simulink library "HANcoder_STM32_Target"  (R2018a)
settings: Solver=ode45  StartTime=0.0  StopTime=10.0  RelTol=1e-3  EnableMultiTasking=on
libraries: simulink x3
(part 1 of 7)
settings Model: Creator=HANcoder  LastModifiedBy=tatzs
settings Model: ModifiedHistory=|
  | la_obwlf -- Thu Sep 01 12:12:55 2016 -- Version 0.33
  | 
  | 
  | 
  | 
  | 
  | 
  | la_obwlf -- Thu Sep 01 09:23:34 2016 -- Version 0.33
  | changed the version in the Base Sample Time block
  | 
  | 
  | 
  | la_obwlf -- Tue Aug 30 15:48:17 2016 -- Version 0.33
settings DataIOCC: LimitDataPoints=on  SaveFormat=Array  SignalLoggingSaveFormat=ModelDataLogs
settings OptimizationCC: ExpressionDepthLimit=2147483647  LifeSpan=inf
settings DebuggingCC: UnderspecifiedInitializationDetection=Classic  MergeDetectMultiDrivingBlocksExec=none  SolverPrmCheckMsg=warning  FcnCallInpInsideContextMsg=warning  StateNameClashWarn=warning  SFUnexpectedBacktrackingDiag=warning  SFNoUnconditionalDefaultTransitionDiag=warning  SFExecutionAtInitializationDiag=none
settings HardwareCC: ProdBitPerPointer=32  ProdBitPerSizeT=32  ProdBitPerPtrDiffT=32  ProdLargestAtomicFloat=None  ProdIntDivRoundTo=Undefined  ProdEndianess=Unspecified  ProdWordSize=32  ProdHWDeviceType=32-bit Generic
settings ModelReferenceCC: PropagateSignalLabelsOutOfModel=off
settings CodeAppCC: StateflowObjectComments=on
settings GRTTargetCC: TargetLangStandard=C89/C90 (ANSI)  GeneratePreprocessorConditionals=Disable all  CombineOutputUpdateFcns=off  GRTInterface=on
settings ConfigComp: CovMetricSettings=dw  CovHtmlReporting=on  CovSaveCumulativeToWorkspaceVar=on  CovSaveSingleToWorkspaceVar=on  CovExternalEMLEnable=off

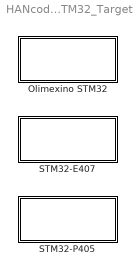
== system HANcoder_STM32_Target ==
  Olimexino STM32 : Subsystem
      settings: MoveFcn=drawLogos
      mask Display:
      | disp('Olimexino STM32')
      | patch([80 86 86],[8 14 2],[1 0 0]);patch([88 88 94],[14 2 8],[0 0 0.35]);
  STM32-E407 : Subsystem
      settings: MoveFcn=drawLogos
      mask Display:
      | disp('STM32-E407')
      | patch([80 86 86],[8 14 2],[1 0 0]);patch([88 88 94],[14 2 8],[0 0 0.35]);
  STM32-P405 : Subsystem
      settings: MoveFcn=drawLogos
      mask Display:
      | disp('STM32-P405')
      | patch([80 86 86],[8 14 2],[1 0 0]);patch([88 88 94],[14 2 8],[0 0 0.35]);

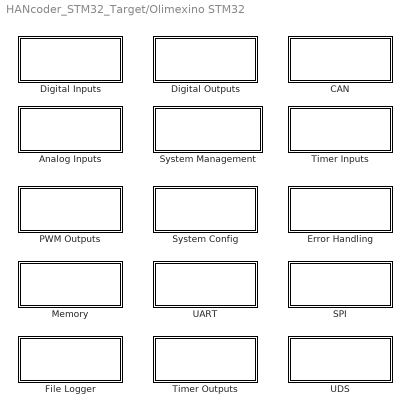
== system HANcoder_STM32_Target/Olimexino STM32 ==
  Analog Inputs : Subsystem
      settings: MoveFcn=drawLogos
      mask Display: fprintf('Analog Inputs');patch([85 91 91],[8 14 2],[1 0 0]);patch([93 93 99],[14 2 8],[0 0 0.35]);
  CAN : Subsystem
      settings: MoveFcn=drawLogos
      mask Display: fprintf('CAN');patch([85 91 91],[8 14 2],[1 0 0]);patch([93 93 99],[14 2 8],[0 0 0.35]);
  Digital Inputs : Subsystem
      settings: MoveFcn=drawLogos
      mask Display: fprintf('Digital Inputs');patch([85 91 91],[8 14 2],[1 0 0]);patch([93 93 99],[14 2 8],[0 0 0.35]);
  Digital Outputs : Subsystem
      settings: MoveFcn=drawLogos
      mask Display: fprintf('Digital Outputs');patch([85 91 91],[8 14 2],[1 0 0]);patch([93 93 99],[14 2 8],[0 0 0.35]);
  Error Handling : Subsystem
      settings: MoveFcn=drawLogos
      mask Display: fprintf('Error Handling');patch([85 91 91],[8 14 2],[1 0 0]);patch([93 93 99],[14 2 8],[0 0 0.35]);
  File Logger : Subsystem
      settings: MoveFcn=drawLogos
      mask Display: fprintf('File Logger');patch([85 91 91],[8 14 2],[1 0 0]);patch([93 93 99],[14 2 8],[0 0 0.35]);
  Memory : Subsystem
      settings: MoveFcn=drawLogos
      mask Display: fprintf('Memory');patch([85 91 91],[8 14 2],[1 0 0]);patch([93 93 99],[14 2 8],[0 0 0.35]);
  PWM Outputs : Subsystem
      settings: MoveFcn=drawLogos
      mask Display: fprintf('PWM Outputs');patch([85 91 91],[8 14 2],[1 0 0]);patch([93 93 99],[14 2 8],[0 0 0.35]);
  SPI : Subsystem
      settings: MoveFcn=drawLogos
      mask Display: fprintf('SPI');patch([85 91 91],[8 14 2],[1 0 0]);patch([93 93 99],[14 2 8],[0 0 0.35]);
  System Config : Subsystem  RequirementInfo={} %GIDa_b102142c_ec72_4a3a_aedf_acb717d0b820
      settings: MoveFcn=drawLogos
      mask Display: fprintf('System Config');patch([85 91 91],[8 14 2],[1 0 0]);patch([93 93 99],[14 2 8],[0 0 0.35]);
  System Management : Subsystem
      settings: MoveFcn=drawLogos
      mask Display: fprintf('System Management');patch([90 96 96],[8 14 2],[1 0 0]);patch([98 98 104],[14 2 8],[0 0 0.35]);
  Timer Inputs : Subsystem
      settings: MoveFcn=drawLogos
      mask Display: fprintf('Timer Inputs');patch([85 91 91],[8 14 2],[1 0 0]);patch([93 93 99],[14 2 8],[0 0 0.35]);
  Timer Outputs : Subsystem
      settings: MoveFcn=drawLogos
      mask Display: fprintf('Timer Outputs');patch([85 91 91],[8 14 2],[1 0 0]);patch([93 93 99],[14 2 8],[0 0 0.35]);
  UART : Subsystem
      settings: MoveFcn=drawLogos
      mask Display: fprintf('UART');patch([85 91 91],[8 14 2],[1 0 0]);patch([93 93 99],[14 2 8],[0 0 0.35]);
  UDS : Subsystem
      settings: MoveFcn=drawLogos
      mask Display: fprintf('UDS');patch([85 91 91],[8 14 2],[1 0 0]);patch([93 93 99],[14 2 8],[0 0 0.35]);

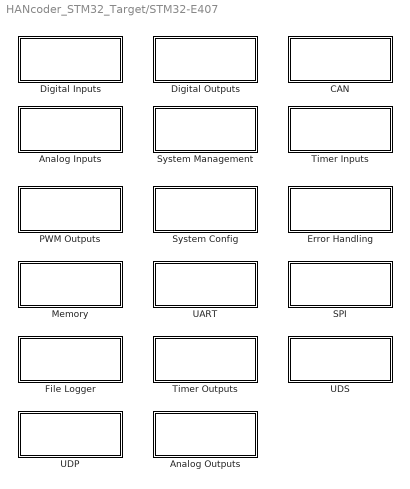
== system HANcoder_STM32_Target/STM32-E407 ==
  Analog Inputs : Subsystem
      settings: MoveFcn=drawLogos
      mask Display: fprintf('Analog Inputs');patch([85 91 91],[8 14 2],[1 0 0]);patch([93 93 99],[14 2 8],[0 0 0.35]);
  Analog Outputs : Subsystem
      settings: MoveFcn=drawLogos
      mask Display: fprintf('Analog Outputs');patch([85 91 91],[8 14 2],[1 0 0]);patch([93 93 99],[14 2 8],[0 0 0.35]);
  CAN : Subsystem
      settings: MoveFcn=drawLogos
      mask Display: fprintf('CAN');patch([85 91 91],[8 14 2],[1 0 0]);patch([93 93 99],[14 2 8],[0 0 0.35]);
  Digital Inputs : Subsystem
      settings: MoveFcn=drawLogos
      mask Display: fprintf('Digital Inputs');patch([85 91 91],[8 14 2],[1 0 0]);patch([93 93 99],[14 2 8],[0 0 0.35]);
  Digital Outputs : Subsystem
      settings: MoveFcn=drawLogos
      mask Display: fprintf('Digital Outputs');patch([85 91 91],[8 14 2],[1 0 0]);patch([93 93 99],[14 2 8],[0 0 0.35]);
  Error Handling : Subsystem
      settings: MoveFcn=drawLogos
      mask Display: fprintf('Error Handling');patch([85 91 91],[8 14 2],[1 0 0]);patch([93 93 99],[14 2 8],[0 0 0.35]);
  File Logger : Subsystem
      settings: MoveFcn=drawLogos
      mask Display: fprintf('File Logger');patch([85 91 91],[8 14 2],[1 0 0]);patch([93 93 99],[14 2 8],[0 0 0.35]);
  Memory : Subsystem
      settings: MoveFcn=drawLogos
      mask Display: fprintf('Memory');patch([85 91 91],[8 14 2],[1 0 0]);patch([93 93 99],[14 2 8],[0 0 0.35]);
  PWM Outputs : Subsystem
      settings: MoveFcn=drawLogos
      mask Display: fprintf('PWM Outputs');patch([85 91 91],[8 14 2],[1 0 0]);patch([93 93 99],[14 2 8],[0 0 0.35]);
  SPI : Subsystem
      settings: MoveFcn=drawLogos
      mask Display: fprintf('SPI');patch([85 91 91],[8 14 2],[1 0 0]);patch([93 93 99],[14 2 8],[0 0 0.35]);
  System Config : Subsystem  RequirementInfo={} %GIDa_b102142c_ec72_4a3a_aedf_acb717d0b820
      settings: MoveFcn=drawLogos
      mask Display: fprintf('System Config');patch([85 91 91],[8 14 2],[1 0 0]);patch([93 93 99],[14 2 8],[0 0 0.35]);
  System Management : Subsystem
      settings: MoveFcn=drawLogos
      mask Display: fprintf('System Management');patch([85 91 91],[8 14 2],[1 0 0]);patch([93 93 99],[14 2 8],[0 0 0.35]);
  Timer Inputs : Subsystem
      settings: MoveFcn=drawLogos
      mask Display: fprintf('Timer Inputs');patch([85 91 91],[8 14 2],[1 0 0]);patch([93 93 99],[14 2 8],[0 0 0.35]);
  Timer Outputs : Subsystem
      settings: MoveFcn=drawLogos
      mask Display: fprintf('Timer Outputs');patch([85 91 91],[8 14 2],[1 0 0]);patch([93 93 99],[14 2 8],[0 0 0.35]);
  UART : Subsystem
      settings: MoveFcn=drawLogos
      mask Display: fprintf('UART');patch([85 91 91],[8 14 2],[1 0 0]);patch([93 93 99],[14 2 8],[0 0 0.35]);
  UDP : Subsystem
      settings: MoveFcn=drawLogos
      mask Display: fprintf('UDP');patch([85 91 91],[8 14 2],[1 0 0]);patch([93 93 99],[14 2 8],[0 0 0.35]);
  UDS : Subsystem
      settings: MoveFcn=drawLogos
      mask Display: fprintf('UDS');patch([85 91 91],[8 14 2],[1 0 0]);patch([93 93 99],[14 2 8],[0 0 0.35]);

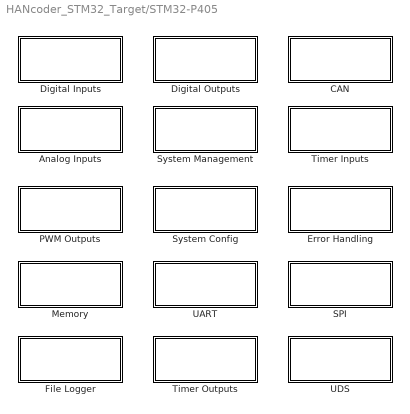
== system HANcoder_STM32_Target/STM32-P405 ==
  Analog Inputs : Subsystem
      settings: MoveFcn=drawLogos
      mask Display: fprintf('Analog Inputs');patch([85 91 91],[8 14 2],[1 0 0]);patch([93 93 99],[14 2 8],[0 0 0.35]);
  CAN : Subsystem
      settings: MoveFcn=drawLogos
      mask Display: fprintf('CAN');patch([85 91 91],[8 14 2],[1 0 0]);patch([93 93 99],[14 2 8],[0 0 0.35]);
  Digital Inputs : Subsystem
      settings: MoveFcn=drawLogos
      mask Display: fprintf('Digital Inputs');patch([85 91 91],[8 14 2],[1 0 0]);patch([93 93 99],[14 2 8],[0 0 0.35]);
  Digital Outputs : Subsystem
      settings: MoveFcn=drawLogos
      mask Display: fprintf('Digital Outputs');patch([85 91 91],[8 14 2],[1 0 0]);patch([93 93 99],[14 2 8],[0 0 0.35]);
  Error Handling : Subsystem
      settings: MoveFcn=drawLogos
      mask Display: fprintf('Error Handling');patch([85 91 91],[8 14 2],[1 0 0]);patch([93 93 99],[14 2 8],[0 0 0.35]);
  File Logger : Subsystem
      settings: MoveFcn=drawLogos
      mask Display: fprintf('File Logger');patch([85 91 91],[8 14 2],[1 0 0]);patch([93 93 99],[14 2 8],[0 0 0.35]);
  Memory : Subsystem
      settings: MoveFcn=drawLogos
      mask Display: fprintf('Memory');patch([85 91 91],[8 14 2],[1 0 0]);patch([93 93 99],[14 2 8],[0 0 0.35]);
  PWM Outputs : Subsystem
      settings: MoveFcn=drawLogos
      mask Display: fprintf('PWM Outputs');patch([85 91 91],[8 14 2],[1 0 0]);patch([93 93 99],[14 2 8],[0 0 0.35]);
  SPI : Subsystem
      settings: MoveFcn=drawLogos
      mask Display: fprintf('SPI');patch([85 91 91],[8 14 2],[1 0 0]);patch([93 93 99],[14 2 8],[0 0 0.35]);
  System Config : Subsystem  RequirementInfo={} %GIDa_b102142c_ec72_4a3a_aedf_acb717d0b820
      settings: MoveFcn=drawLogos
      mask Display: fprintf('System Config');patch([85 91 91],[8 14 2],[1 0 0]);patch([93 93 99],[14 2 8],[0 0 0.35]);
  System Management : Subsystem
      settings: MoveFcn=drawLogos
      mask Display: fprintf('System Management');patch([85 91 91],[8 14 2],[1 0 0]);patch([93 93 99],[14 2 8],[0 0 0.35]);
  Timer Inputs : Subsystem
      settings: MoveFcn=drawLogos
      mask Display: fprintf('Timer Inputs');patch([85 91 91],[8 14 2],[1 0 0]);patch([93 93 99],[14 2 8],[0 0 0.35]);
  Timer Outputs : Subsystem
      settings: MoveFcn=drawLogos
      mask Display: fprintf('Timer Outputs');patch([85 91 91],[8 14 2],[1 0 0]);patch([93 93 99],[14 2 8],[0 0 0.35]);
  UART : Subsystem
      settings: MoveFcn=drawLogos
      mask Display: fprintf('UART');patch([85 91 91],[8 14 2],[1 0 0]);patch([93 93 99],[14 2 8],[0 0 0.35]);
  UDS : Subsystem
      settings: MoveFcn=drawLogos
      mask Display: fprintf('UDS');patch([85 91 91],[8 14 2],[1 0 0]);patch([93 93 99],[14 2 8],[0 0 0.35]);

== system HANcoder_STM32_Target/Olimexino STM32/Analog Inputs ==
  Analog Input : Subsystem  Tag=HANcoder_TARGET_STM32_Olimexino  mask(Analog Input){pinID=CON2 - A0, tsamp=-1, filtered=off}
      mask prompts: pinID "Input pin"; tsamp "Sample time"; filtered "Use oversampling and filtering (causes high CPU load)"
      mask help:
      | Function
      | ========
      | Reads the analog/digital conversion results of an analog input pin.
      |
      | Parameters
      | ==========
      | Input pin:
      |   Selects the analog input to read
      |
      | Outport
      | ==========
      | uint16 12-bit conversion results (0-4095).
      mask init:
      | pinIDInfoStr = sfcn_analog_in_mcb(1, pinID, 0);
      settings: MoveFcn=drawLogos
      mask Help: web('sfcn_analog_in.html');
      mask TypeOptions pinID: CON2 - A0 | CON2 - A1 | CON2 - A2 | CON2 - A3 | CON2 - A4 | CON2 - A5 | CON3 - D0 | CON3 - D1 | CON3 - D2 | CON3 - D3/LED2 | CON4 - D10 | CON4 - D11 | CON4 - D12 | CON4 - D13/LED1 | EXT - D27 | EXT - D28
      mask Display: fprintf('Analog Input\n%s', pinIDInfoStr);patch([135 141 141],[8 14 2],[1 0 0]);patch([143 143 149],[14 2 8],[0 0 0.35]);

== system HANcoder_STM32_Target/Olimexino STM32/CAN ==
  CAN : Subsystem
      settings: MoveFcn=drawLogos
      mask Display: fprintf('CAN');patch([85 91 91],[8 14 2],[1 0 0]);patch([93 93 99],[14 2 8],[0 0 0.35]);
  CANopenClient : Subsystem
      settings: MoveFcn=drawLogos
      mask Display: fprintf('CANopenClient');patch([85 91 91],[8 14 2],[1 0 0]);patch([93 93 99],[14 2 8],[0 0 0.35]);
  CANopenNode : Subsystem
      settings: MoveFcn=drawLogos
      mask Display: fprintf('CANopenNode');patch([85 91 91],[8 14 2],[1 0 0]);patch([93 93 99],[14 2 8],[0 0 0.35]);

== system HANcoder_STM32_Target/Olimexino STM32/Digital Inputs ==
  Digital Input : Subsystem  Tag=HANcoder_TARGET_STM32_Olimexino  mask(Digital Input){pinID=CON2 - A0, config=Pulldown, tsamp=-1}
      mask prompts: pinID "Input pin"; config "Configuration"; tsamp "Sample time"
      mask help:
      | Function
      | ========
      | Reads the state of a digital input pin.
      |
      | Parameters
      | ==========
      | Input pin:
      |   Selects the digital input to read
      | Configuration:
      |   Determines if the input is floating or is connected to an internal
      |   pull-up or pull-down resistor.
      |
      | Outport
      | ==========
      | State of the pin. 0 means logical low and 1 logical high
      mask init:
      | pinIDInfoStr = sfcn_digital_in_mcb(1, pinID, config);
      settings: MoveFcn=drawLogos
      mask Help: web('sfcn_digital_in.html');
      mask TypeOptions pinID: CON2 - A0 | CON2 - A1 | CON2 - A2 | CON2 - A3 | CON2 - A4 | CON2 - A5 | CON3 - D0 | CON3 - D1 | CON3 - D2 | CON3 - D3/LED2 | CON3 - D4 | CON3 - D5 - 5V Tolerant | CON3 - D6 - 5V Tolerant | CON3 - D7 - 5V Tolerant | CON4 - D8 - 5V Tolerant | CON4 - D9 - 5V Tolerant | CON4 - D10 | CON4 - D11 | CON4 - D12 | CON4 - D13/LED1 | EXT - D25 - 5V Tolerant | EXT - D26 - 5V Tolerant | EXT - D29 - 5V Tolerant | EXT - D30 - 5V Tolerant | EXT - D31 - 5V Tolerant | EXT - D32 - 5V Tolerant | EXT - D33 - 5V Tolerant | EXT - D34 - 5V Tolerant | EXT - D35 - 5V Tolerant | EXT - D36 - 5V Tolerant | EXT - D37 - 5V Tolerant | Pushbutton - BUT/BOOT0 - 5V Tolerant
      mask TypeOptions config: Floating | Pullup | Pulldown
      mask Display: fprintf('Digital Input\n%s', pinIDInfoStr);patch([135 141 141],[8 14 2],[1 0 0]);patch([143 143 149],[14 2 8],[0 0 0.35]);

== system HANcoder_STM32_Target/Olimexino STM32/Digital Outputs ==
  Digital Output : Subsystem  Tag=HANcoder_TARGET_STM32_Olimexino  mask(Digital Output){pinID=CON2 - A0, config=Push pull, tsamp=-1}
      mask prompts: pinID "Output pin"; config "Configuration"; tsamp "Sample time"
      mask help:
      | Function
      | ========
      | Controls the state of a digital output pin.
      |
      | Parameters
      | ==========
      | Output pin:
      |   Selects the digital output to control
      | Configuration:
      |   Open drain (output float when digital high) or push-pull (output connected
      |   to Vcc when digital high).
      |
      | Inport
      | ==========
      | State of the pin. 0 means logical low and 1 logical high
      mask init:
      | pinIDInfoStr = sfcn_digital_out_mcb(1, pinID, config);
      settings: CopyFcn=sfcn_digital_out_chk();  MoveFcn=drawLogos
      mask Help: web('sfcn_digital_out.html');
      mask TypeOptions pinID: CON2 - A0 | CON2 - A1 | CON2 - A2 | CON2 - A3 | CON2 - A4 | CON2 - A5 | CON3 - D0 | CON3 - D1 | CON3 - D2 | CON3 - D3/LED2 | CON3 - D4 | CON3 - D5 | CON3 - D6 | CON3 - D7 | CON4 - D8 | CON4 - D9 | CON4 - D10 | CON4 - D11 | CON4 - D12 | CON4 - D13/LED1 | EXT - D25 | EXT - D26 | EXT - D31 | EXT - D32 | EXT - D35 | EXT - D36 | EXT - D37
      mask Callback pinID: sfcn_digital_out_chk();
      mask TypeOptions config: Open drain | Push pull
      mask Display: fprintf('Digital Output\n%s', pinIDInfoStr);patch([135 141 141],[8 14 2],[1 0 0]);patch([143 143 149],[14 2 8],[0 0 0.35]);

== system HANcoder_STM32_Target/Olimexino STM32/Error Handling ==
  Clear errors : Subsystem  Tag=HANcoder_TARGET_STM32_Olimexino  mask(Clear errors){eepromString=Active}
      mask prompts: eepromString "Active or Stored error"
      mask help:
      | [Function]
      | Clears the active(RAM) or stored(EEPROM) errors.
      |
      | [Triggerport]
      | Connect the port to a trigger source to execute the block only when necessary.
      mask init:
      | sfcn_controller_error_clearerrors_mcb(eepromString)
      settings: MoveFcn=drawLogos
      mask Help: web('sfcn_controller_error_clearerrors.html');
      mask TypeOptions eepromString: Active | Stored
      mask Display: fprintf('Clear %s Errors', eepromString);patch([80 86 86],[8 14 2],[1 0 0]);patch([88 88 94],[14 2 8],[0 0 0.35]);
  Delete error : Subsystem  Tag=HANcoder_TARGET_STM32_Olimexino  mask(Delete error){useInPorts=off, errorID=hex2dec('8000'), para=10}
      mask prompts: useInPorts "Use inports"; errorID "Error code"; para "Error parameter"
      mask help:
      | [Function]
      | Delete an error defined by error code and parameter
      | from RAM.
      | Error ID and parameter can be specified in the mask or with inports.
      |
      | [Parameters]
      | Error code
      | Error parameter
      |
      | [Inputs]
      | 1 - Error code [uint16]
      | 2 - Error parameter [uint8]
      |
      | [Triggerport]
      | Connect the port to a trigger source to execute the block only when necessary.
      mask init:
      | sfcn_controller_error_deleteerror_mcb(useInPorts, errorID, para)
      settings: MoveFcn=drawLogos
      mask Help: web('sfcn_controller_error_deleteerror.html');
      mask Display: fprintf('Delete error');patch([80 86 86],[8 14 2],[1 0 0]);patch([88 88 94],[14 2 8],[0 0 0.35]);
  Read active error : Subsystem  Tag=HANcoder_TARGET_STM32_Olimexino  mask(Read active error){tsamp=-1}
      mask prompts: tsamp "Sample time"
      mask help:
      | Function
      | ==========
      | Read an active error from RAM.
      |
      | Inport
      | ==========
      | Input is the number of the error in the error list, which can be 1..64. UINT8
      |
      | Outports
      | ==========
      | 1: UINT8 - total amount of errors.
      | 2: UINT16 - error code.
      | 3: UINT8  - error parameter.
      | 4: UINT8  - occurrence count.
      | 5: UINT32 - last occurrence time since startup [milliseconds].
      |
      | Note that the requested error was set and read only if occurrence count > 0.
      mask init:
      | sfcn_controller_error_readerror_mcb(0)
      settings: MoveFcn=drawLogos
      mask Help: web('sfcn_controller_error_readerror.html');
      mask Display: fprintf('Read active error');patch([80 86 86],[8 14 2],[1 0 0]);patch([88 88 94],[14 2 8],[0 0 0.35]);
  Read stored error : Subsystem  Tag=HANcoder_TARGET_STM32_Olimexino  mask(Read stored error){tsamp=-1}
      mask prompts: tsamp "Sample time"
      mask help:
      | Function
      | ==========
      | Read a stored error from EEPROM.
      |
      | Inport
      | ==========
      | Input is the number of the error in the error list, which can be 1..64. UINT8
      |
      | Outports
      | ==========
      | 1: UINT8 - total amount of errors.
      | 2: UINT16 - error code.
      | 3: UINT8  - error parameter.
      | 4: UINT8  - occurrence count.
      | 5: UINT32 - last occurrence time since startup [milliseconds].
      |
      | Note that the requested error was set and read only if occurrence count > 0.
      mask init:
      | sfcn_controller_error_readerror_mcb(1)
      settings: MoveFcn=drawLogos
      mask Help: web('sfcn_controller_error_readerror.html');
      mask Display: fprintf('Read stored error');patch([80 86 86],[8 14 2],[1 0 0]);patch([88 88 94],[14 2 8],[0 0 0.35]);
  Search active error : Subsystem  Tag=HANcoder_TARGET_STM32_Olimexino  mask(Search active error){tsamp=-1}
      mask prompts: tsamp "Sample time"
      mask help:
      | Function
      | ==========
      | Searches for the erorr with the specified error Code and Param in RAM.
      |
      | Inport
      | ==========
      | 1: UINT16 - Error Code
      | 2: UINT8   - Error Parameter
      |
      | Outports
      | ==========
      | 1: UINT8   - occurrence count.
      | 2: UINT32 - last occurrence time since startup [milliseconds]
      |
      | Note that when occurrence count equals zero, the error is not found.
      mask init:
      | sfcn_controller_error_searcherror_mcb(0)
      settings: MoveFcn=drawLogos
      mask Help: web('sfcn_controller_error_searcherror.html');
      mask Display: fprintf('Search active error');patch([80 86 86],[8 14 2],[1 0 0]);patch([88 88 94],[14 2 8],[0 0 0.35]);
  Search stored error : Subsystem  Tag=HANcoder_TARGET_STM32_Olimexino  mask(Search stored error){tsamp=-1}
      mask prompts: tsamp "Sample time"
      mask help:
      | Function
      | ==========
      | Searches for the erorr with the specified error Code and Param in EEPROM.
      |
      | Inport
      | ==========
      | 1: UINT16 - Error Code
      | 2: UINT8   - Error Parameter
      |
      | Outports
      | ==========
      | 1: UINT8   - occurrence count.
      | 2: UINT32 - last occurrence time since startup [milliseconds]
      |
      | Note that when occurrence count equals zero, the error is not found.
      mask init:
      | sfcn_controller_error_searcherror_mcb(1)
      settings: MoveFcn=drawLogos
      mask Help: web('sfcn_controller_error_searcherror.html');
      mask Display: fprintf('Search stored error');patch([80 86 86],[8 14 2],[1 0 0]);patch([88 88 94],[14 2 8],[0 0 0.35]);
  "Store error " : Subsystem  Tag=HANcoder_TARGET_STM32_Olimexino  mask(Store error){useInPorts=off, errorCode=hex2dec('8000'), parameter=10}
      mask prompts: useInPorts "Use inports"; errorCode "Error code"
      mask help:
      | [Function]
      | Store an error to RAM (and EEPROM if new) of the controller.
      | Error ID and parameter can be specified in the mask or with inports.
      |
      | [Parameters]
      | Error code
      | Error parameter
      |
      | [Inputs]
      | 1 - Error code [uint16]
      | 2 - Error parameter [uint8]
      |
      | [Triggerport]
      | Connect the port to a trigger source to execute the block only when necessary.
      mask init:
      | sfcn_controller_error_storeerror_in_mcb(useInPorts, errorCode, parameter, 1)
      settings: MoveFcn=drawLogos
      mask Help: web('sfcn_controller_error_storeerror.html');
      mask Display: fprintf('Store error');patch([80 86 86],[8 14 2],[1 0 0]);patch([88 88 94],[14 2 8],[0 0 0.35]);
  Total Errors : Subsystem  Tag=HANcoder_TARGET_STM32_Olimexino  mask(Total active or stored errors){eepromString=Active, tsamp=-1}
      mask prompts: eepromString "Active or Stored error"; tsamp "Sample time"
      mask help:
      | [Function]
      | Returns the total amount of active or stored errors
      |
      | [Parameters]
      | Active or Stored error [-]
      | sampleTime: [s]
      |
      | [Outputs]
      | Port 1 :Total number of errors [uint8]
      | Port 2 :Highest occuring severity [uint8]
      mask init:
      | sfcn_controller_error_totalerrors_mcb(eepromString, tsamp);
      settings: MoveFcn=drawLogos
      mask Help: web('sfcn_controller_error_totalerrors.html');
      mask TypeOptions eepromString: Active | Stored
      mask Display: fprintf('Total %s Errors', eepromString);patch([80 86 86],[8 14 2],[1 0 0]);patch([88 88 94],[14 2 8],[0 0 0.35]);

== system HANcoder_STM32_Target/Olimexino STM32/File Logger ==
  File Logger Close : Subsystem  Tag=HANcoder_TARGET_STM32_Olimexino  mask(File Logger Close){}
      mask help:
      | Function
      | ========
      | With the File Logger module active, the data values of the configured signals
      | are sampled at a fixed time interval and written to the log-file on the SD-card.
      |
      | The log-file needs to be explicitly closed at the end of a logging session for the
      | log-file to actually appear on the SD-card.
      |
      | Ideally, this block is called during software shutdown for example when the ignition
      | signal goes low in automotive applications. An external trigger can also be used such
      | as a button press event or CAN message reception.
      |
      | Triggerport
      | ===========
      | Connect the port to a trigger source to execute the block only when necessary.
      mask init:
      | sfcn_filelogger_close_mcb();
      settings: MoveFcn=drawLogos
      mask Help: web('sfcn_filelogger_close.html')
      mask Display: fprintf('File Logger Close');patch([80 86 86],[8 14 2],[1 0 0]);patch([88 88 94],[14 2 8],[0 0 0.35]);
  File Logger Init : Subsystem  Tag=HANcoder_TARGET_STM32_Olimexino  mask(File Logger Init){filename='mylog.txt', autoincrement=on, firstline='time;signal1;signal2;signal3', interval=100, maxsignals=3, dotseparator=off, autostart=on}
      mask prompts: autoincrement "Add auto-incrementing number to filename"; firstline "First line in log-file"; interval "Logging interval (ms)"; maxsignals "Maximum signals to log"; dotseparator "Use dot-character as decimal separator (comma otherwise)"; autostart "Automatically start logging"
      mask help:
      | Function
      | ==========
      | Initializes the File Logger module.
      |
      | Parameters per channel
      | ======================
      | - Specify filename for the log-file
      | - Select if a 3-digit auto-incrementing number should be added to the log-file
      | - Specify the first line in the log-file
      | - Specify the logging interval in milliseconds
      | - Specify the maximum number of signals to log
      | - Select if a comma or dot should be used a the decimal point in numbers
      | - Select if logging should automatically start after initialization. If not then
      |   a trigger input will appear that can be used to trigger the logging start.
      mask init:
      | sfcn_filelogger_init_mcb(filename, firstline, interval, maxsignals, dotseparator, autoincrement, autostart);
      settings: MoveFcn=drawLogos
      mask Help: web('sfcn_filelogger_init.html')
      mask Display: fprintf('File Logger Init');patch([95 101 101],[8 14 2],[1 0 0]);patch([103 103 109],[14 2 8],[0 0 0.35]);
  File Logger Signal : Subsystem  Tag=HANcoder_TARGET_STM32_Olimexino  mask(File Logger Signal){signalIdx=0, dataType=uint8}
      mask prompts: signalIdx "Signal Index"; dataType "Signal Data Type"
      mask help:
      | Function
      | ==========
      | Configures the signal to be logged by the File Logger module.
      |
      | Parameters per channel
      | ======================
      | - Specify the zero based index of the signal for the File Logger module. In the
      |   File Logger Init block the maximum number of signals was configured
      |   (max_signals). Valid values for this paramter are 0..(max_signals-1).
      | - Select the data type of the signal.
      mask init:
      | sfcn_filelogger_signal_mcb(signalIdx, dataType);
      settings: MoveFcn=drawLogos
      mask Help: web('sfcn_filelogger_signal.html')
      mask TypeOptions dataType: double | single | int8 | uint8 | int16 | uint16 | int32 | uint32
      mask Display: fprintf('File Logger Signal\n(Index %d)', signalIdx);patch([95 101 101],[8 14 2],[1 0 0]);patch([103 103 109],[14 2 8],[0 0 0.35]);

== system HANcoder_STM32_Target/Olimexino STM32/Memory ==
  EEPROM : Subsystem
      settings: MoveFcn=drawLogos
      mask Display: fprintf('EEPROM');patch([85 91 91],[8 14 2],[1 0 0]);patch([93 93 99],[14 2 8],[0 0 0.35]);

== system HANcoder_STM32_Target/Olimexino STM32/PWM Outputs ==
  PWM Duty Cycle : Subsystem  Tag=HANcoder_TARGET_STM32_Olimexino  mask(Pulse Width Modulation Set Duty Cycle){pinID=TIM1 - CON3 - D6, tsamp=-1}
      mask prompts: pinID "Output pin"; tsamp "Sample time"
      mask help:
      | Function
      | ========
      | A 'PWM Duty Cycle' block allows the duty cycle of the generated PWM signal to
      | changed.
      | Note that this only works properly if a 'PWM Init' block is also present
      | for initializing the related PWM module.
      |
      | Parameters
      | ==========
      | PWM pin:
      |   Selects the PWM pin for which the duty cycle should be updated.
      |
      | Inport
      | ==========
      | uint16 10-bit unsigned value (0..1023) to represent the duty cycle (0..100%) for
      | each enabled channel.
      mask init:
      | pinIDInfoStr = sfcn_pwmout_setduty_mcb(1, pinID);
      settings: MoveFcn=drawLogos
      mask Help: web('sfcn_pwmout_setduty.html');
      mask TypeOptions pinID: TIM1 - CON3 - D6 | TIM1 - CON3 - D7 | TIM1 - CON4 - D8 | TIM2 - CON3 - D2 | TIM2 - CON3 - D3 | TIM2 - CON3 - D0 | TIM3 - EXT - D35 | TIM3 - EXT - D36 | TIM3 - EXT - D37 | TIM4 - CON3 - D5 | TIM4 - CON4 - D9 | TIM4 - CON4 - D14 | TIM4 - EXT - D24
      mask Display: fprintf('PWM Set Duty Cycle\n%s', pinIDInfoStr);patch([135 141 141],[8 14 2],[1 0 0]);patch([143 143 149],[14 2 8],[0 0 0.35]);
  PWM Init : Subsystem  Tag=HANcoder_TARGET_STM32_Olimexino  mask(Pulse Width Modulation Initialization){moduleID=TIM1: D6 & D7 & D8 & n/a + N-channels D32 & D33 & D34, frequency=1004, alignment=Edge aligned, enableIRQoutput=off, ch1On=off, ch1Pol=Active high, ch1Inv=off, ch2On=off, ch2Pol=Active high, ch2Inv=off, ch3On=off, ch3Pol=Active high, ch3Inv=off, ch4On=off, ch4Pol=Active high, ch4Inv=off}
      mask prompts: moduleID "PWM module"; frequency "Signal frequency [Hz]"; alignment "Signal alignment"; enableIRQoutput "Enable IRQ output"; ch1On "Generate PWM signal on channel 1"; ch1Pol "Select signal polarity"; ch1Inv "Enable inverted signal on additional output pin"; ch2On "Generate PWM signal on channel 2"; ch2Pol "Select signal polarity"; ch2Inv "Enable inverted signal on additional output pin"; ch3On "Generate PWM signal on channel 3"; ch3Pol "Select signal polarity"; ch3Inv "Enable inverted signal on additional output pin"; ch4On "Generate PWM signal on channel 4"; ch4Pol "Select signal polarity"; ch4Inv "Enable inverted signal on additional output pin"
      mask help:
      | Function
      | ========
      | A 'PWM Init' block configures one of the STM32 timer modules for PWM
      | functionality, allowing a PWM signal to be generated on up to 4 timer
      | channels and their associated output pins.
      |
      | Parameters
      | ==========
      | General - PWM module:
      |   Select the PWM module to use. The name in the combo box contains
      |   information about which pins on the target belong to this timer module.
      |   Also the first pin corresponds with the first channel and so on:
      |   TIMx: Ch1 & Ch2 & Ch3...
      |
      | General - Signal frequency:
      |   Determines the signal frequency in Hz. If you click 'Apply' after entering
      |   the desired frequency it will automatically be adjusted to the closest
      |   supported value.
      |
      | General - Signal Aligment:
      |   Determines the aligment of the signal. It can either be edge aligned or
      |   center aligned.
      |
      | General - Enable IRQ output
      |   Controls whether or not the IRQ output is available.
      |
      | Channel x - Generate PWM signal on channel x:
      |   Enable to configure the channel for PWM functionality so that the PWM signal
      |   is outputted on the channel's associated microcontroller pin.
      |
      | Channel x - Signal polarity:
      |   Selects the polarity of the signal.
      |
      | Channel x - Enable inverted signal on additional output pin:
      |   When enabled, a second PWM signal will be generated on an additional
      |   microcontroller pin where the signal is an exact inversion of the first signal.
      mask init:
      | moduleIDInfoStr = sfcn_pwmout_init_mcb(1, moduleID, frequency, alignment, enableIRQoutput, ch1On, ch2On, ch3On, ch4On, ch1Pol, ch2Pol, ch3Pol, ch4Pol, ch1Inv, ch2Inv, ch3Inv, ch4Inv);
      settings: CopyFcn=sfcn_pwmout_init_chk();  MoveFcn=drawLogos
      mask Help: web('sfcn_pwmout_init.html');
      mask TypeOptions moduleID: TIM1: D6 & D7 & D8 & n/a + N-channels D32 & D33 & D34  | TIM2: D2 & D3 & n/a & D0 | TIM3: D35 & D36 & D37 & n/a | TIM4: D5 & D9 & D14 & D24
      mask Callback moduleID: sfcn_pwmout_init_chk();
      mask TypeOptions alignment: Edge aligned | Center aligned
      mask TypeOptions ch1Pol: Active high | Active low
      mask TypeOptions ch2Pol: Active high | Active low
      mask TypeOptions ch3Pol: Active high | Active low
      mask TypeOptions ch4Pol: Active high | Active low
      mask Display: fprintf('PWM Init\n%s', moduleIDInfoStr);patch([220 226 226],[8 14 2],[1 0 0]);patch([228 228 234],[14 2 8],[0 0 0.35]);

== system HANcoder_STM32_Target/Olimexino STM32/SPI ==
  SPI master init : Subsystem  Tag=HANcoder_TARGET_STM32_Olimexino  mask(SPI master init){channel=SPI1: D13 & D12 & D11, speed=9000 kHz, polarity=Idle low, phase=Sample bit on 1st clock edge}
      mask prompts: speed "Communication speed"
      mask help:
      | Function
      | ==========
      | Initialized a SPI master channel.
      |
      | Parameters per channel
      | ======================
      | - Select channel (SCK MISO MOSI)
      | - Select communication speed
      | - Select clock signal polarity
      | - Select clock phase to sample a bit
      mask init:
      | spiChannelInfoStr = sfcn_spi_master_init_mcb(1, channel, speed, polarity, phase);
      settings: CopyFcn=sfcn_spi_master_init_chk();  MoveFcn=drawLogos
      mask Help: web('sfcn_spi_master_init.html')
      mask TypeOptions channel: SPI1: D13 & D12 & D11 | SPI2: D32 & D33 & D34
      mask Callback channel: sfcn_spi_master_init_chk();
      mask TypeOptions speed: 36000 kHz | 18000 kHz | 9000 kHz | 4500 kHz | 2250 kHz | 1125 kHz | 562.5 kHz | 281.25 kHz
      mask TypeOptions polarity: Idle low | Idle high
      mask TypeOptions phase: Sample bit on 1st clock edge | Sample bit on 2nd clock edge
      mask Display: fprintf('SPI master init\n%s', spiChannelInfoStr);patch([211 217 217],[8 14 2],[1 0 0]);patch([219 219 225],[14 2 8],[0 0 0.35]);
  SPI master transfer : Subsystem  Tag=HANcoder_TARGET_STM32_Olimexino  mask(SPI master transfer){channel=SPI1: D13 & D12 & D11, useSS=off, SSpin=CON2 - A0, SSenable=on, SSdisable=on, delayCycles=0, tsamp=-1}
      mask prompts: useSS "Use slave select output"; SSpin "Slave select output pin"; SSenable "Enable slave select before transfer"; SSdisable "Disable slave select after transfer"; delayCycles "Delay cycles between slave select enable and transfer"; tsamp "Sample time"
      mask help:
      | Function
      | ==========
      | Performs a byte transfer via SPI.
      |
      | Parameters per channel
      | ======================
      | - Select channel
      | - Select if a Slave Select output should be controlled
      |   * Select the Slave Select digital output pin
      |   * Select if the Slave Select should be made logic low before the transfer
      |   * Select if the Slave Select should be made logic high after the transfer
      |   * Enter the number of CPU cycles to delay between Slave Select enable and the transfer
      |
      | Inputs
      | ======
      | The byte value to send to the slave.
      |
      | Outputs
      | =======
      | The byte value received from the slave.
      mask init:
      | spiChannelInfoStr = sfcn_spi_master_transfer_mcb(1, channel, useSS, SSpin, SSenable, SSdisable, delayCycles);
      settings: MoveFcn=drawLogos
      mask Help: web('sfcn_spi_master_transfer.html')
      mask TypeOptions channel: SPI1: D13 & D12 & D11 | SPI2: D32 & D33 & D34
      mask TypeOptions SSpin: CON2 - A0 | CON2 - A1 | CON2 - A2 | CON2 - A3 | CON2 - A4 | CON2 - A5 | CON3 - D0 | CON3 - D1 | CON3 - D2 | CON3 - D3/LED2 | CON3 - D4 | CON3 - D5 | CON3 - D6 | CON3 - D7 | CON4 - D8 | CON4 - D9 | CON4 - D10 | CON4 - D11 | CON4 - D12 | CON4 - D13/LED1 | EXT - D25 | EXT - D26 | EXT - D31 | EXT - D32 | EXT - D35 | EXT - D36 | EXT - D37
      mask Display: fprintf('SPI master transfer\n%s', spiChannelInfoStr);patch([210 216 216],[8 14 2],[1 0 0]);patch([218 218 224],[14 2 8],[0 0 0.35]);

== system HANcoder_STM32_Target/Olimexino STM32/System Config ==
  Base Sample Time config : Subsystem  Tag=HANcoder_TARGET_STM32_Olimexino  Description=HANcoder Target STM32-Olimexino blockset version 0.5  mask(Base Sample Time config){baseSampleTime=10, extraStack=25}
      mask prompts: baseSampleTime "Define the base sample time [ms]"; extraStack "Additional task stack (bytes):"
      mask help:
      | Function
      | ==========
      | Sets the Base Sample Time in the model, and automatically sets the sample
      | time in the solver step time menu when the model is simulated or build.
      |
      | Parameters
      | ==========
      | Base Sample Time [milliseconds]
      | Default:    10[ms]
      | Min:        0.1[ms]
      |
      | Note: This is the only block where sample time is set in miliseconds,
      | all other blocks work with sample time in seconds
      |
      | It is possible to reserve extra stack space for the OS task that executes
      | the model on the embedded target (AppCtrlTask).
      mask init:
      | sfcn_base_sample_time_mcb(baseSampleTime*1000, extraStack,1);
      | HANcoderStruct = get_param(gcb,'UserData');
      | BlocksetVersion = HANcoderStruct.BlocksetVersion;
      settings: MoveFcn=drawLogos
      mask Help: web('sfcn_base_sample_time.html')
      mask Display: fprintf('Blockset version %s\nBase Sample Time:\n %gms',BlocksetVersion,baseSampleTime);patch([91 97 97],[8 14 2],[1 0 0]);patch([99 99 105],[14 2 8],[0 0 0.35]);
  Build settings : Subsystem  Tag=HANcoder_TARGET_STM32_Olimexino  mask(Build Settings){AutoASAP2add=on, AutoFlash=USB}
      mask prompts: AutoASAP2add "Add signals and parameters automatically"; AutoFlash "Automatic flash after build"
      mask help:
      | Function
      | ==========
      | Auto Add:
      | Here you can turn the automatic adding of Signals and Parameters on or off. If the option is on all the parameters and signals which are not defined in the workspace will be added. You will be prompted for the value.
      |
      | Auto Flash:
      | This option will automatically start MicroBoot with the selected interface.
      settings: MoveFcn=drawLogos
      mask Help: web('build_settings.html')
      mask TypeOptions AutoASAP2add: on | off
      mask TypeOptions AutoFlash: off | USB | CAN
      mask DialogControl ParameterTabVar0 Prompt: Auto Add
      mask DialogControl Control3 Prompt: With this option the undefined parameters and signals will automatically be added to the workspace for use with HANtune. You will be prompted for the parameter values.
      mask DialogControl ParameterTabVar01 Prompt: Auto Flash
      mask DialogControl Control2 Prompt: With this option you can choose to automatically start MicroBoot after the build is complete. MicroBoot will start flashing using the selected interface.
      mask Display: fprintf('Build settings\nAuto Add: %s\nAuto Flash: %s',AutoASAP2add, AutoFlash);patch([114 120 120],[8 14 2],[1 0 0]);patch([122 122 128],[14 2 8],[0 0 0.35]);
  CAN config : Subsystem  Tag=HANcoder_TARGET_STM32_Olimexino  mask(CAN config){canBus1=on, baudRate1=500, rxMask1=hex2dec('00000000'), rxCode1=hex2dec('00000000'), rxMode1=Receive only 11-bit message identifiers, txBufSize1=32, evBufSize1=32}
      mask prompts: canBus1 "Use CAN bus"; baudRate1 "Baudrate CAN bus [kbit/s]"; rxMask1 "Reception filter Mask CAN bus"; rxCode1 "Reception filter Code CAN bus"; rxMode1 "Reception filter Mode CAN bus"; txBufSize1 "Transmit buffer size CAN bus (max 256)"; evBufSize1 "Event buffer size CAN bus"
      mask help:
      | Function
      | ==========
      | Configures the settings for the STM32's CAN busses.
      |
      | Parameters per channel
      | ======================
      | - Activate channel
      | - Select baud rate (default 500[kbit/s])
      | - Select reception acceptance filter Code
      | - Select reception acceptance filter Mask
      | - Select reception acceptance filter Mode
      mask init:
      | sfcn_can_config_mcb(txBufSize1, evBufSize1, canBus1, baudRate1, rxMask1, rxCode1, rxMode1, 0, 1, 0, 0, 1);
      settings: MoveFcn=drawLogos
      mask Help: web('sfcn_can_config.html')
      mask TypeOptions baudRate1: 125 | 250 | 500 | 1000
      mask TypeOptions rxMode1: Receive only 11-bit message identifiers | Receive only 29-bit message identifiers | Received both 11- and 29-bit message identifiers
      mask Display: fprintf('CAN1 : %x',canBus1);patch([58 64 64],[8 14 2],[1 0 0]);patch([66 66 72],[14 2 8],[0 0 0.35]);
  Custom ID config : Subsystem  Tag=HANcoder_TARGET_STM32_Olimexino  mask(Custom ID config){softID=softwareID, softNUM=1}
      mask prompts: softID "Software ID Name"; softNUM "Software Version Number"
      mask help:
      | Function:
      | =========
      | This block can be used to override the generated software ID as the current software version which is used for identification purposes.
      | It can also be used to add a version number behind the software ID.
      |
      | Details:
      | ========
      | If only a software version number is filled in, a software ID will be generated and the version number will be placed behind it.
      | Atleast one pf the fields has to be filled in.
      |
      | Parameters:
      | ===========
      | Software ID name:
      | Fill in the desired custom ID. Must fit in a UINT8
      | Software Version Number:
      | Fill in the desired version number. Must fit in a UINT8
      mask init:
      | sfcn_custom_version_config_mcb(softID, softNUM)
      settings: MoveFcn=drawLogos
      mask Help: web('sfcn_custom_ID_config.html')
      mask Display: fprintf('Custom software ID:\n "%s"\n Software version:\n "%s"', char(softID), char(softNUM));patch([112 118 118],[8 14 2],[1 0 0]);patch([120 120 126],[14 2 8],[0 0 0.35]);
  XCP on CAN config : Subsystem  Tag=HANcoder_TARGET_STM32_Olimexino  mask(XCP on CAN config){canBus=CAN 1, croID=hex2dec('665'), dtoID=hex2dec('666')}
      mask prompts: canBus "CAN channel"; croID "CRO identifier"; dtoID "DTO identifier"
      mask help:
      | Function
      | ==========
      | Implements XCP communication into your application.
      |
      | Parameter
      | ==========
      | Specify the CAN channel to be used for XCP.
      | Specify the CAN CRO message identifier for XCP (master->slave).
      | Specify the CAN DTO message identifier for XCP (slave->master).
      |
      | Notes
      | ==========
      | Baudrates can be modified in the CAN config block.
      mask init:
      | sfcn_can_xcp_config_mcb(canBus, croID, dtoID)
      settings: MoveFcn=drawLogos
      mask Help: web('sfcn_can_xcp_config.html')
      mask TypeOptions canBus: CAN 1
      mask Display: fprintf('XCP over CAN: %x',canBus);patch([69 75 75],[8 14 2],[1 0 0]);patch([77 77 83],[14 2 8],[0 0 0.35]);
  XCP on USB config : Subsystem  Tag=HANcoder_TARGET_STM32_Olimexino  mask(XCP on USB config){}
      mask help:
      | Function
      | ==========
      | Implements XCP communication into your application using the USB Virtual COM-port.
      mask init:
      | sfcn_usb_xcp_config_mcb()
      settings: MoveFcn=drawLogos
      mask Help: web('sfcn_usb_xcp_config.html')
      mask Display: fprintf('XCP over USB');patch([69 75 75],[8 14 2],[1 0 0]);patch([77 77 83],[14 2 8],[0 0 0.35]);

== system HANcoder_STM32_Target/Olimexino STM32/System Management ==
  Enter Critical Section : Subsystem  Tag=HANcoder_TARGET_STM32_Olimexino  mask(Enter a critical section){tsamp=-1}
      mask prompts: tsamp "Sample time"
      mask help:
      | Function
      | ==========
      | Enters a critical section that can not be interrupted. This block must
      | always be used in a pair together with "Exit Critical Section". Click the
      | Help-button for a detailed example on how to use this block.
      mask init:
      | sfcn_critical_enter_mcb();
      settings: MoveFcn=drawLogos
      mask Help: web('sfcn_critical_section.html');
      mask Display: fprintf('Enter Critical Section');patch([95 101 101],[8 14 2],[1 0 0]);patch([103 103 109],[14 2 8],[0 0 0.35]);
  Exit Critical Section : Subsystem  Tag=HANcoder_TARGET_STM32_Olimexino  mask(Exit a critical section){tsamp=-1}
      mask prompts: tsamp "Sample time"
      mask help:
      | Function
      | ==========
      | Exits a critical section. This block must always be used in a pair together
      | with "Enter Critical Section". Click the Help-button for a detailed example
      | on how to use this block.
      mask init:
      | sfcn_critical_exit_mcb();
      settings: MoveFcn=drawLogos
      mask Help: web('sfcn_critical_section.html');
      mask Display: fprintf('Exit Critical Section');patch([95 101 101],[8 14 2],[1 0 0]);patch([103 103 109],[14 2 8],[0 0 0.35]);
  Get CPU load : Subsystem  Tag=HANcoder_TARGET_STM32_Olimexino  mask(Get CPU load){mode=Current CPU load, tsamp=-1}
      mask prompts: tsamp "Sample time"
      mask help:
      | Function
      | ==========
      | Get the CPU load of the system.
      |
      | Parameters
      | ==========
      | Mode specifies if the current CPU load should be read or the maximum CPU
      | load since reset.
      |
      | Outport
      | ==========
      | CPU load as a percentage.
      mask init:
      | if mode==1
      |   modeStr = 'current';
      | else
      |   modeStr = 'maximum';
      | end
      | sfcn_controller_cpu_getload_mcb(mode);
      settings: MoveFcn=drawLogos
      mask Help: web('sfcn_controller_cpu_getload.html');
      mask TypeOptions mode: Current CPU load | Maximum CPU load
      mask Display: fprintf('Get %s\nCPU load', modeStr);patch([95 101 101],[8 14 2],[1 0 0]);patch([103 103 109],[14 2 8],[0 0 0.35]);
  Get free Heap : Subsystem  Tag=HANcoder_TARGET_STM32_Olimexino  mask(Get free Heap){tsamp=-1}
      mask prompts: tsamp "Sample time"
      mask help:
      | Function
      | ==========
      | Obtains the number of bytes that are still available on the heap.
      |
      | Outport
      | ==========
      | Number of bytes that are still available on the heap.
      mask init:
      | sfcn_controller_getheap_mcb();
      settings: MoveFcn=drawLogos
      mask Help: web('sfcn_controller_getheap.html');
      mask Display: fprintf('Get free Heap');patch([95 101 101],[8 14 2],[1 0 0]);patch([103 103 109],[14 2 8],[0 0 0.35]);
  Get free Stack : Subsystem  Tag=HANcoder_TARGET_STM32_Olimexino  mask(Get free Stacl){taskIdx=Application Control Task, tsamp=-1}
      mask prompts: taskIdx "Task name"; tsamp "Sample time"
      mask help:
      | Function
      | ========
      | Obtains the number of bytes that are still available on the stack of a particular task.
      |
      | Parameter
      | =========
      | Name of the task for which the free stack space should be read.
      |
      | Outport
      | =======
      | Number of bytes that are still available on the task's stack.
      mask init:
      | sfcn_controller_getstack_mcb(taskIdx);
      settings: MoveFcn=drawLogos
      mask Help: web('sfcn_controller_getstack.html');
      mask TypeOptions taskIdx: Idle Task | Timer Task | Can Event Task | Can Transmit Task | Application Control Task
      mask Display: fprintf('Get free Stack');patch([95 101 101],[8 14 2],[1 0 0]);patch([103 103 109],[14 2 8],[0 0 0.35]);
  Reset ECU : Subsystem  Tag=HANcoder_TARGET_STM32_Olimexino  mask(Reset ECU){}
      mask help:
      | Function
      | ==========
      | Triggering this block causes the ECU to reset.
      mask init:
      | sfcn_controller_reset_mcb()
      settings: MoveFcn=drawLogos
      mask Help: web('sfcn_controller_reset.html');
      mask Display: fprintf('Reset ECU');patch([60 66 66],[8 14 2],[1 0 0]);patch([68 68 74],[14 2 8],[0 0 0.35]);
